simulink model "controllerForJoints"  (R2019a)
settings: Solver=VariableStepAuto  StartTime=0.0  StopTime=4  RelTol=1e-3
values from neighbouring files (symbols this model uses):
  b = 3.5077E-6    (= 3.5077e-06)    [constant_values.m]
  J = 3.2284E-6    (= 3.2284e-06)    [constant_values.m]
  K = 0.0274    [constant_values.m]
  L = 2.75E-6    (= 2.75e-06)    [constant_values.m]
  R = 4    [constant_values.m]
libraries: simulink x4
settings Model: Creator=Mustafa  LastModifiedBy=Mustafa

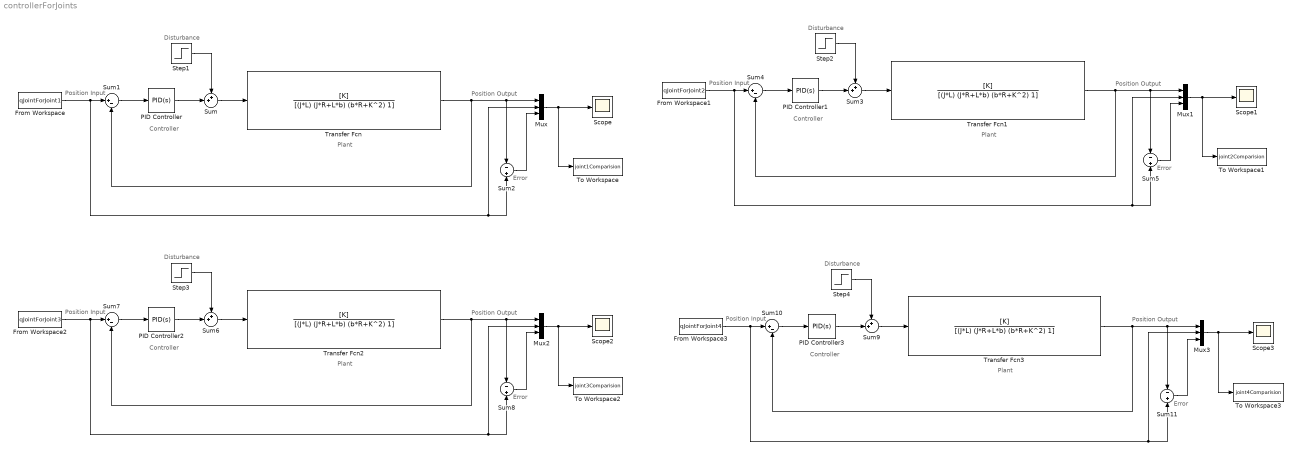
== system controllerForJoints ==
  note: Error
  note: Plant
  note: Controller
  note: Disturbance
  note: Position Output
  note: Position Input
  note: Plant
  note: Disturbance
  note: Position Output
  note: Error
  note: Position Input
  note: Controller
  note: Plant
  note: Disturbance
  note: Position Output
  note: Disturbance
  note: Controller
  note: Error
  note: Position Output
  note: Error
  note: Position Input
  note: Position Input
  note: Controller
  note: Plant
  From Workspace : FromWorkspace  VariableName=qJointForJoint1  SampleTime=0.02
  From Workspace1 : FromWorkspace  VariableName=qJointForJoint2  SampleTime=0.02
  From Workspace2 : FromWorkspace  VariableName=qJointForJoint3  SampleTime=0.02
  From Workspace3 : FromWorkspace  VariableName=qJointForJoint4  SampleTime=0.02
  Mux{,1..3} (4 alike) : Mux  Inputs=3
  PID Controller{,1..3} (4 alike) : simulink/Continuous/PID Controller  Controller=PID  Form=Parallel  TimeDomain=Continuous-time  SampleTime=-1  IntegratorMethod=Forward Euler  FilterMethod=Forward Euler  ControllerParametersSource=internal  P=324.104063209864  I=32186.2687929709  D=0.578196525659438  UseFilter=on  N=154690.014365904  TunerSelectOption=Transfer Function Based (PID Tuner App)  InitialConditionSource=internal  InitialConditionForIntegrator=0  InitialConditionForFilter=0  DifferentiatorICPrevScaledInput=0  ExternalReset=none  TrackingMode=off  Kt=1  LimitOutput=off  UpperSaturationLimit=inf  LowerSaturationLimit=-inf  LinearizeAsGain=on  AntiWindupMode=none  Kb=1  POutMin=[]  POutMax=[]  IOutMin=[]  IOutMax=[]  DOutMin=[]  DOutMax=[]  NOutMin=[]  NOutMax=[]  SumOutMin=[]  SumOutMax=[]  SaturationOutMin=[]  SaturationOutMax=[]  PParamMin=[]  PParamMax=[]  IParamMin=[]  IParamMax=[]  DParamMin=[]  DParamMax=[]  NParamMin=[]  NParamMax=[]  KbParamMin=[]  KbParamMax=[]  KtParamMin=[]  KtParamMax=[]  KbOutMin=[]  KbOutMax=[]  KtOutMin=[]  KtOutMax=[]  IntegratorOutMin=[]  IntegratorOutMax=[]  FilterOutMin=[]  FilterOutMax=[]  SumI1OutMin=[]  SumI1OutMax=[]  SumI2OutMin=[]  SumI2OutMax=[]  SumI3OutMin=[]  SumI3OutMax=[]  SumI4OutMin=[]  SumI4OutMax=[]  SumDOutMin=[]  SumDOutMax=[]  DifferentiatorOutMin=[]  DifferentiatorOutMax=[]  FilterDiffOutCoefMin=[]  FilterDiffOutCoefMax=[]  ReciprocalOutMin=[]  ReciprocalOutMax=[]  SumDenOutMin=[]  SumDenOutMax=[]  SumNumOutMin=[]  SumNumOutMax=[]  DivideOutMin=[]  DivideOutMax=[]  IntegratorContinuousStateAttributes=''  IntegratorStateMustResolveToSignalObject=off  IntegratorRTWStateStorageClass=Auto  FilterContinuousStateAttributes=''  FilterStateMustResolveToSignalObject=off  FilterRTWStateStorageClass=Auto  ParallelPVariant=InternalParameters  IdealPVariant=Disabled  IVariant=InternalParameters  DVariant=InternalParameters  IntegratorVariant=Continuous  SatVariant=Disabled  AWVariant=Passthrough  PCopyVariant=Disabled  TRVariant=Disabled  FdbkBlocksVariant=Forward  IdealPFdbkVariant=Disabled  SatFdbkVariant=Disabled  DerivativeFilterVariant=ContFilter  NVariant=InternalParameters  NCopyVariant=Disabled  FilterICVariant=InternalICsFilter  IntegratorICVariant=InternalICs  ExternalResetVariant=Disabled  TRSumVariant=Passthrough  SumFdbkVariant=Disabled  SumVariant=Sum_PID
  Scope{,1..3} (4 alike) : Scope
  Step{1..4} (4 alike) : Step  Time=0  SampleTime=0
  Sum{,3,6,9} (4 alike) : Sum  Inputs=++|
  Sum{1,4,7,10} (4 alike) : Sum  Inputs=|+-
  Sum{2,5,8,11} (4 alike) : Sum  Inputs=-|+
  To Workspace : ToWorkspace  VariableName=joint1Comparision  SaveFormat=Timeseries  SampleTime=-1
  To Workspace1 : ToWorkspace  VariableName=joint2Comparision  SaveFormat=Timeseries  SampleTime=-1
  To Workspace2 : ToWorkspace  VariableName=joint3Comparision  SaveFormat=Timeseries  SampleTime=-1
  To Workspace3 : ToWorkspace  VariableName=joint4Comparision  SaveFormat=Timeseries  SampleTime=-1
  Transfer Fcn{,1..3} (4 alike) : TransferFcn  Numerator=[K]  Denominator=[(J*L) (J*R+L*b) (b*R+K^2) 1]
  wires:
  PID Controller/1 -> Sum/2
  Sum/1 -> Transfer Fcn/1
  Transfer Fcn/1 -> Mux/1, Sum2/1, Sum1/2
  Sum1/1 -> PID Controller/1
  Step1/1 -> Sum/1
  From Workspace/1 -> Sum2/2, Mux/2, Sum1/1
  Mux/1 -> To Workspace/1, Scope/1
  Sum2/1 -> Mux/3
  Mux1/1 -> To Workspace1/1, Scope1/1
  From Workspace1/1 -> Sum5/2, Mux1/2, Sum4/1
  Sum5/1 -> Mux1/3
  Step2/1 -> Sum3/1
  PID Controller1/1 -> Sum3/2
  Transfer Fcn1/1 -> Mux1/1, Sum5/1, Sum4/2
  Sum3/1 -> Transfer Fcn1/1
  Sum4/1 -> PID Controller1/1
  Mux2/1 -> To Workspace2/1, Scope2/1
  From Workspace2/1 -> Sum8/2, Mux2/2, Sum7/1
  Sum8/1 -> Mux2/3
  Step3/1 -> Sum6/1
  Transfer Fcn2/1 -> Mux2/1, Sum8/1, Sum7/2
  Sum6/1 -> Transfer Fcn2/1
  Transfer Fcn3/1 -> Mux3/1, Sum11/1, Sum10/2
  Sum10/1 -> PID Controller3/1
  Sum9/1 -> Transfer Fcn3/1
  PID Controller2/1 -> Sum6/2
  Step4/1 -> Sum9/1
  From Workspace3/1 -> Sum11/2, Mux3/2, Sum10/1
  Sum11/1 -> Mux3/3
  Sum7/1 -> PID Controller2/1
  Mux3/1 -> To Workspace3/1, Scope3/1
  PID Controller3/1 -> Sum9/2
